simulink model "Iek1"  (Simulink 5.0)
settings: Solver=FixedStepDiscrete  StartTime=0.0  StopTime=10000000.0  RelTol=1e-3
libraries: simulink x2
settings Model: Creator=scaife  LastModifiedBy=scaife  ExtModeAutoUpdateStatusClock=off

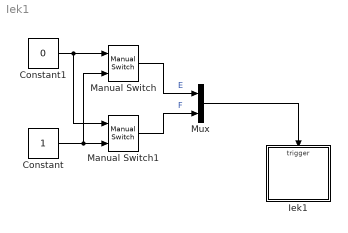
== system Iek1 ==
  Constant : Constant
  Constant1 : Constant  Value=0
  Iek1 : Stateflow chart
  Manual Switch : simulink/Signal Routing/Manual Switch  sw=1  action=0
  Manual Switch1 : simulink/Signal Routing/Manual Switch  sw=1  action=0
  Mux : Mux  Inputs=2
  wires:
  Constant1/1 -> Manual Switch/1, Manual Switch1/1
  Constant/1 -> Manual Switch1/2, Manual Switch/2
  Manual Switch1/1 -> Mux/2  "F"
  Manual Switch/1 -> Mux/1  "E"
  Mux/1 -> Iek1/Trigger

== stateflow chart Iek1 ==
  state T1 [parallel]
    state B
    state A
    (default) -> A
    A -> B : E
    B -> A : E
  state T2 [parallel]
    state C
    state D
    (default) -> C
    D -> C : F
    C -> D : F
  state T3 [parallel]
    state a
    state c
    state b
    state d
    (default) -> a
    a -> c : exit(A)
    c -> d : enter(A)
    d -> b : exit(C)
    b -> a : enter(C)
    c -> b : enter(D)
    b -> c : enter(B)
  events: E input EITHER_EDGE_EVENT; F input EITHER_EDGE_EVENT
